simulink model "c2d_controller"  (R2015a)
settings: Solver=ode45  StartTime=0.0  StopTime=20  FixedStep=0.01  RelTol=1e-3
values from neighbouring files (symbols this model uses):
  Gcz = c2d(Gcs, Ts, 'zoh')    [c2d_controller_m.m]
  Gs = 1.0 / (s * s + 5 * s + 1)    [c2d_controller_m.m]
  simout_sampling_time = 0.01    [c2d_controller_m.m]
  Ts = T0 + step_changes * i    [c2d_controller_m.m]
settings Model: Creator=Xiaotian  LastModifiedBy=Xiaotian

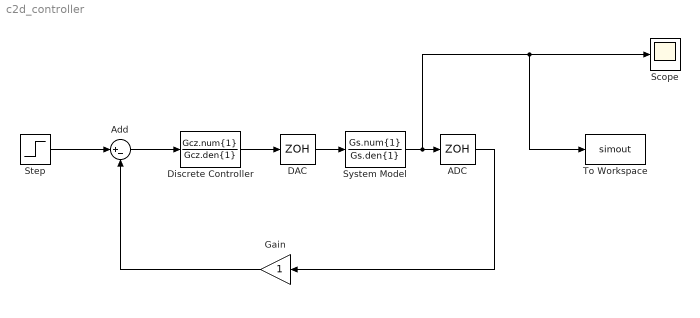
== system c2d_controller ==
  ADC : ZeroOrderHold  SampleTime=Ts
  Add : Sum  Inputs=|+-
  DAC : ZeroOrderHold  SampleTime=Ts
  Discrete Controller : DiscreteTransferFcn  Numerator=Gcz.num{1}  Denominator=Gcz.den{1}  SampleTime=Ts
  Gain : Gain
  Scope : Scope
  Step : Step  Time=0  SampleTime=0
  System Model : TransferFcn  Numerator=Gs.num{1}  Denominator=Gs.den{1}
  To Workspace : ToWorkspace  VariableName=simout  SaveFormat=Timeseries  SampleTime=simout_sampling_time
  wires:
  Gain/1 -> Add/2
  Add/1 -> Discrete Controller/1
  Discrete Controller/1 -> DAC/1
  DAC/1 -> System Model/1
  System Model/1 -> Scope/1, To Workspace/1, ADC/1
  ADC/1 -> Gain/1
  Step/1 -> Add/1
